simulink model "Leg_Sim_VariableDamping"  (R2020b)
settings: Solver=ode23s  StartTime=0.0  StopTime=1  RelTol=1e-3
values from neighbouring files (symbols this model uses):
  body = Leg_Pars_Body    [Leg_Script_Powered.m]    (also in Leg_Script_Socket_VariableDamping.m; Leg_Script_VariableDamping.m)
  ctrl = Leg_Pars_Ctrl_Powered    [Leg_Script_Powered.m]    (also in Leg_Script_Socket_VariableDamping.m = Leg_Pars_Ctrl_VariableDamping; Leg_Script_VariableDamping.m = Leg_Pars_Ctrl_VariableDamping)
  device = Leg_Pars_Device_Powered    [Leg_Script_Powered.m]    (also in Leg_Script_Socket_VariableDamping.m = Leg_Pars_Device_VariableDamping; Leg_Script_VariableDamping.m = Leg_Pars_Device_VariableDamping)
  FD = [1;1;0;1;1;0;0;1]    [Leg_Script_Powered.m]    (also in Leg_Script_Socket_VariableDamping.m = [1;1;0;1;1;1;1;0;0;1]; Leg_Script_VariableDamping.m)
  human = Leg_Pars_Human(body)    [Leg_Script_Powered.m]    (also in Leg_Script_Socket_VariableDamping.m; Leg_Script_VariableDamping.m)
  intent = [0;1;0]    [Leg_Script_Powered.m]    (also in Leg_Script_Socket_VariableDamping.m; Leg_Script_VariableDamping.m)
  intentv = [1.1;1.1;0.8]    [Leg_Script_Powered.m]    (also in Leg_Script_Socket_VariableDamping.m = [1.1; 1.1; 1.4; 1.4; 1.1; 1.1; 1.4;0.8]; Leg_Script_VariableDamping.m = [1.1; 1.1; 1.4; 1.4; 1.1; 1.1; 1.4;0.8])
  q0 = [0;1;ref.pt_walk ... (first row only)    [Leg_Script_Powered.m]    (also in Leg_Script_Socket_VariableDamping.m; Leg_Script_VariableDamping.m)
  qd0 = [intentv(1)*1.2*intent(1);0;0;0;0;0;0;0]    [Leg_Script_Powered.m]    (also in Leg_Script_Socket_VariableDamping.m = [intentv(1)*1.25*intent(1);0;0;0;0;0;0;0;0;0]; Leg_Script_VariableDamping.m)
  robsim = robotcell2mat(robot)    [Leg_Script_Powered.m]    (also in Leg_Script_Socket_VariableDamping.m; Leg_Script_VariableDamping.m)
  t_intent = [0;1;15]    [Leg_Script_Powered.m]    (also in Leg_Script_Socket_VariableDamping.m = [0;1;35]; Leg_Script_VariableDamping.m = [0;1;35])
  t_intentv = [0;10;15]    [Leg_Script_Powered.m]    (also in Leg_Script_Socket_VariableDamping.m = [0; 9.99; 10; 14.99; 15; 20; 25;35]; Leg_Script_VariableDamping.m = [0; 9.99; 10; 14.99; 15; 20; 25;35])
  u0 = zeros(1,length(robot.gc.body))    [Leg_Script_Powered.m]    (also in Leg_Script_Socket_VariableDamping.m; Leg_Script_VariableDamping.m)
undefined symbols (not defined in the file or in its folder): syst
libraries: simulink x4
(part 1 of 2)
settings Model: Creator=JDriessen  LastModifiedBy=jdriessen
settings SolverCC: ZeroCrossAlgorithm=Adaptive
settings DebuggingCC: MaskedZcDiagnostic=none  IgnoredZcDiagnostic=none

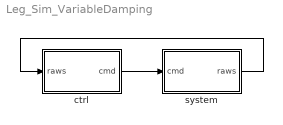
== system Leg_Sim_VariableDamping ==
  ctrl : Subsystem
  system : Subsystem
  wires:
  system/1(raws) -> ctrl/1(raws)
  ctrl/1(cmd) -> system/1(cmd)

== system Leg_Sim_VariableDamping/ctrl ==
  raws : Inport
  Clock : Clock
      settings: Decimation=3
  High-level ctrl : Subsystem  mask{fsm=ctrl.fsm}
      mask prompts: fsm "FSM Parameters"
      mask help: High-level control: Finite State Machine (FSM)
  Mid-level ctrl : Subsystem  mask{mid=ctrl.mid}
      mask prompts: mid "Mid-level controller parameters"
      mask help: Mid-level control
      mask DialogControl Container2 Prompt: Parameters
  Signal processing : Subsystem  mask{pre=ctrl.pre}
      mask prompts: pre "Signal processing parameters"
      mask help: Signal processing
  clock : ToWorkspace  VariableName=t_ctrl  SampleTime=ctrl.t_step
      settings: Save2DSignal=2-D array (concatenate along first dimension)
  cmd : Outport
  wires:
  raws/1 -> Signal processing/1(raws)
  Mid-level ctrl/1(cmd) -> cmd/1
  High-level ctrl/1(state) -> Mid-level ctrl/2(state)
  Clock/1 -> clock/1
  Signal processing/2(tube) -> High-level ctrl/2(tube)
  Signal processing/1(knee) -> High-level ctrl/1(knee), Mid-level ctrl/1(knee)

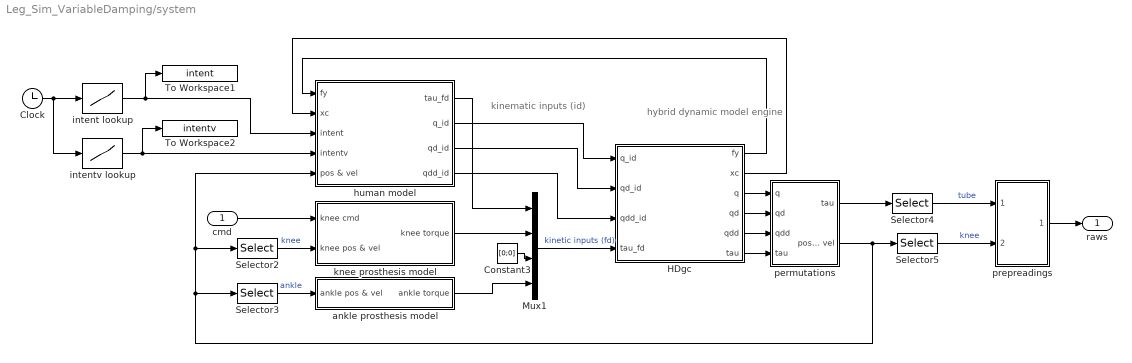
== system Leg_Sim_VariableDamping/system ==
  note: kinematic inputs (id)
  note: hybrid dynamic
      | model engine
  cmd : Inport
  Clock : Clock
  Constant3 : Constant  Value=[0;0]
  HDgc : Subsystem  mask{model=robsim, fd=FD, q0=q0, qd0=qd0, u0=u0}
      mask prompts: model "robot structure"; fd "joint dynamics type logic (1=forward, 0=inverse)"; q0 "initial joint position (forward dynamics)"; qd0 "initial joint velocities (forward dynamics)"; u0 "initial ground contact deformations"
      mask help: Hybrid dynamics engine with ground contact model.
      mask init:
      | fdd = fd~=0; % convert to logical (if not already)
      | i_fd = find(fd); % indices fd joints
      | model.fd_i = cumsum(fd); % joint index assign array fd joints
      | model.NB_fd = sum(fd); % number of fd joints
      | i_id = find(~fd); % indices id joints
      | model.id_i = cumsum(~fd); % joint index assign array id joints
      | model.NB_id = sum(~fd); % number of id joints
      | model.ND = size(model.Xtree(:,:,1),1); % 3 = planar, 6 = spatial
      | model.S = zeros(model.ND,model.NB); % pre-allocate motion subspace matrix
      | for i = 1:model.NB % fill motion subspace matrix
      |     switch model.jtype(i,:)
      |     case 'Rx' % revolute X axis
      |         model.S = [1;0;0;0;0;0];
      |     case 'Ry' % revolute Y axis
      |         model.S = [0;1;0;0;0;0];
      |     case 'Rz' % revolute Z axis
      |         model.S = [0;0;1;0;0;0];
      |     case 'Px' % prismatic X axis
      |         model.S = [0;0;0;1;0;0];
      |     case 'Py' % prismatic Y axis
      |         model.S = [0;0;0;0;1;0];
      |     case 'Pz' % prismatic Z axis
      |         model.S = [0;0;0;0;0;1];
      |     case 'Hz' % helical (Z axis)
      |         model.S = [0;0;1;0;0;jtyp.pars.pitch];
      |     case 'rz' % planar revolute
      |         model.S(:,i) = [1;0;0];
      |     case 'px'% planar prismatic X axis
      |         model.S(:,i) = [0;1;0];
      |     case 'py'% planar prismatic Y axis
      |         model.S(:,i) = [0;0;1];
      |     otherwise
      |         error( 'unrecognised joint code ''%s''', code );
      |     end
      | end
      | % gravity
      | g = model.gravity;
      | if model.ND == 3		% is model planar?
      |     model.a_grav = [0;g(1);g(2)];
      | else
      |     model.a_grav = [0;0;0;g(1);g(2);g(3)];
      | end
  Mux1 : Mux
  Selector2 : Selector  InputPortWidth=robsim.NB*2  IndexOptions=Index vector (dialog)  Indices=5+[0;robsim.NB]  OutputSizes=1
  Selector3 : Selector  InputPortWidth=robsim.NB*2  IndexOptions=Index vector (dialog)  Indices=8+[0;robsim.NB]  OutputSizes=1
  Selector4 : Selector  InputPortWidth=robsim.NB  IndexOptions=Index vector (dialog)  Indices=[7;6]  OutputSizes=1
  Selector5 : Selector  InputPortWidth=robsim.NB*2  IndexOptions=Index vector (dialog)  Indices=5  OutputSizes=1
  To Workspace1 : ToWorkspace  VariableName=intent  SampleTime=-1
      settings: Save2DSignal=2-D array (concatenate along first dimension)
  To Workspace2 : ToWorkspace  VariableName=intentv  SampleTime=-1
      settings: Save2DSignal=2-D array (concatenate along first dimension)
  ankle prosthesis model : Subsystem  mask{ank=device.ankle}
      mask prompts: ank "ankle parameters"
      mask help: Ankle Prosthesis Model
  human model : Subsystem  mask{ref=human.ref, imp=human.imp, SLIP=human.SLIP, x_step_0=human.x_step_0, Kthrust_0=human.Kthrust_0, bdy=body, rob=robsim}
      mask prompts: ref "human reference trajectories and parameters"; imp "human impedance parameters"; SLIP "human SLIP parameters"; x_step_0 "initial estimate step length"; Kthrust_0 "initial estimate thrust gain"; bdy "body parameters"; rob "robot structure"
      mask help: Human model
  intent lookup : Lookup_n-D  NumberOfTableDimensions=1  BreakpointsForDimension1=t_intent  IndexSearchMethod=Linear search  Table=intent  InterpMethod=Flat  InternalRulePriority=Speed  RndMeth=Simplest  InputSameDT=on
  intentv lookup : Lookup_n-D  NumberOfTableDimensions=1  BreakpointsForDimension1=t_intentv  IndexSearchMethod=Linear search  Table=intentv  ExtrapMethod=Clip  InternalRulePriority=Speed  RndMeth=Simplest  InputSameDT=on
  knee prosthesis model : Subsystem  mask{dmp=device.knee.damper, ese=device.knee.ext_endstop, esf=device.knee.flx_endstop}
      mask prompts: dmp "knee damper parameters"; ese "knee extension endstop parameters"; esf "knee flexion endstop parameters"
      mask help: Knee Prosthesis Model
  permutations : Subsystem
  prepreadings : Subsystem
  raws : Outport
  wires:
  Mux1/1 -> HDgc/4(tau_fd)  "kinetic inputs (fd)"
  Selector5/1 -> prepreadings/2(knee pos)  "knee"
  Selector4/1 -> prepreadings/1(tube)  "tube"
  Constant3/1 -> Mux1/3
  cmd/1 -> knee prosthesis model/1(knee cmd)
  Selector2/1 -> knee prosthesis model/2(knee pos & vel)  "knee"
  knee prosthesis model/1(knee torque) -> Mux1/2
  Selector3/1 -> ankle prosthesis model/1(ankle pos & vel)  "ankle"
  ankle prosthesis model/1(ankle torque) -> Mux1/4
  HDgc/3(q) -> permutations/1(q)
  HDgc/6(tau) -> permutations/4("tau ")
  permutations/1(tau) -> Selector4/1
  prepreadings/1(raws) -> raws/1
  intent lookup/1 -> human model/3(intent), To Workspace1/1
  permutations/2(pos & vel) -> human model/5(pos & vel), Selector2/1, Selector3/1, Selector5/1
  Clock/1 -> intentv lookup/1, intent lookup/1
  intentv lookup/1 -> human model/4(intentv), To Workspace2/1
  human model/4(qdd_id) -> HDgc/3(qdd_id)
  human model/3(qd_id) -> HDgc/2(qd_id)
  human model/2(q_id) -> HDgc/1(q_id)
  human model/1(tau_fd) -> Mux1/1
  HDgc/1(fy) -> human model/1(fy)
  HDgc/2(xc) -> human model/2(xc)
  HDgc/4(qd) -> permutations/2(qd)
  HDgc/5(qdd) -> permutations/3(qdd)

== system Leg_Sim_VariableDamping/ctrl/High-level ctrl ==
  knee : Inport
  tube : Inport  Port=2
  Chart : Stateflow chart  TreatAsAtomicUnit=on
  Demux : Demux  Outputs=2
  Demux1 : Demux  Outputs=2
  To Workspace : ToWorkspace  VariableName=state  SampleTime=ctrl.t_step
      settings: Save2DSignal=2-D array (concatenate along first dimension)
  To Workspace1 : ToWorkspace  VariableName=tSt  SampleTime=-1
      settings: Save2DSignal=2-D array (concatenate along first dimension)
  To Workspace2 : ToWorkspace  VariableName=tSw  SampleTime=-1
      settings: Save2DSignal=2-D array (concatenate along first dimension)
  state : Outport
  wires:
  Chart/1(state) -> To Workspace/1, state/1
  Demux/2 -> Chart/2(wk)  "pkd"
  Demux/1 -> Chart/1(pk)  "pk"
  knee/1 -> Demux/1
  tube/1 -> Demux1/1
  Demux1/1 -> Chart/3(M)
  Chart/2(tSw) -> To Workspace2/1
  Chart/3(tSt) -> To Workspace1/1
  Demux1/2 -> Chart/4(F)  "F"

== system Leg_Sim_VariableDamping/ctrl/Mid-level ctrl ==
  knee : Inport
  state : Inport  Port=2
  Demux1 : Demux  Outputs=2
  Mid Ctrl : MATLAB Function  Description=Mid-level control  TreatAsAtomicUnit=on  SystemSampleTime=ctrl.t_step
  Terminator2 : Terminator
  To Workspace2 : ToWorkspace  VariableName=cmd_m  SampleTime=-1
      settings: Save2DSignal=2-D array (concatenate along first dimension)
  cmd : Outport
  wires:
  Mid Ctrl/1(cmd_m) -> To Workspace2/1, cmd/1
  state/1 -> Mid Ctrl/2(state)
  knee/1 -> Demux1/1
  Demux1/1 -> Mid Ctrl/1(pk)  "pk"
  Demux1/2 -> Terminator2/1  "pkd"

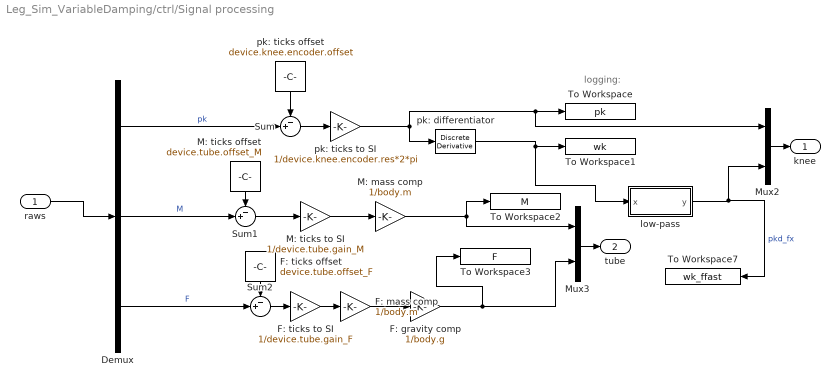
== system Leg_Sim_VariableDamping/ctrl/Signal processing ==
  note: logging:
  raws : Inport
  Demux : Demux  Outputs=3
  F: gravity comp : Gain  Gain=1/body.g
  F: mass comp : Gain  Gain=1/body.m
  F: ticks offset : Constant  Value=device.tube.offset_F
  F: ticks to SI : Gain  Gain=1/device.tube.gain_F
  M: mass comp : Gain  Gain=1/body.m
  M: ticks offset : Constant  Value=device.tube.offset_M
  M: ticks to SI : Gain  Gain=1/device.tube.gain_M
  Mux2 : Mux  Inputs=2
  Mux3 : Mux  Inputs=2
  Sum : Sum  Inputs=-+|
  Sum1 : Sum  Inputs=-+|
  Sum2 : Sum  Inputs=-+|
  To Workspace : ToWorkspace  VariableName=pk  SampleTime=-1
      settings: Save2DSignal=2-D array (concatenate along first dimension)
  To Workspace1 : ToWorkspace  VariableName=wk  SampleTime=-1
      settings: Save2DSignal=2-D array (concatenate along first dimension)
  To Workspace2 : ToWorkspace  VariableName=M  SampleTime=-1
      settings: Save2DSignal=2-D array (concatenate along first dimension)
  To Workspace3 : ToWorkspace  VariableName=F  SampleTime=-1
      settings: Save2DSignal=2-D array (concatenate along first dimension)
  To Workspace7 : ToWorkspace  VariableName=wk_ffast  SampleTime=-1
      settings: Save2DSignal=2-D array (concatenate along first dimension)
  low-pass : Subsystem  mask(1st order Butterworth filter){Wn=pre.freq_fast*ctrl.t_step*2, x0=0, y0=0}
      mask prompts: Wn "cut-off frequency"; x0 "initial condition for previous input"; y0 "initial condition for previous output"
      mask help: The cut-off frequency Wn must be 0.0 < Wn < 1.0, with 1.0 corresponding to half the sample rate.
  pk: differentiator : simulink/Discrete/Discrete Derivative  gainval=1  ICPrevScaledInput=0  OutMin=[]  OutMax=[]  OutDataType=fixdt(1, 16)  OutScaling=2^-10  DoSatur=off
  pk: ticks offset : Constant  Value=device.knee.encoder.offset
  pk: ticks to SI : Gain  Gain=1/device.knee.encoder.res*2*pi
  knee : Outport
  tube : Outport  Port=2
  wires:
  F: gravity comp/1 -> To Workspace3/1, Mux3/2
  F: ticks to SI/1 -> F: mass comp/1
  low-pass/1(y) -> Mux2/2, To Workspace7/1  "pkd_fx"
  Mux3/1 -> tube/1
  pk: ticks to SI/1 -> Mux2/1, To Workspace/1, pk: differentiator/1
  F: mass comp/1 -> F: gravity comp/1
  pk: differentiator/1 -> low-pass/1(x), To Workspace1/1
  M: mass comp/1 -> To Workspace2/1, Mux3/1
  Mux2/1 -> knee/1
  Sum2/1 -> F: ticks to SI/1
  raws/1 -> Demux/1
  F: ticks offset/1 -> Sum2/1
  M: ticks to SI/1 -> M: mass comp/1
  M: ticks offset/1 -> Sum1/1
  Sum/1 -> pk: ticks to SI/1
  Sum1/1 -> M: ticks to SI/1
  pk: ticks offset/1 -> Sum/1
  Demux/1 -> Sum/2  "pk"
  Demux/2 -> Sum1/2  "M"
  Demux/3 -> Sum2/2  "F"

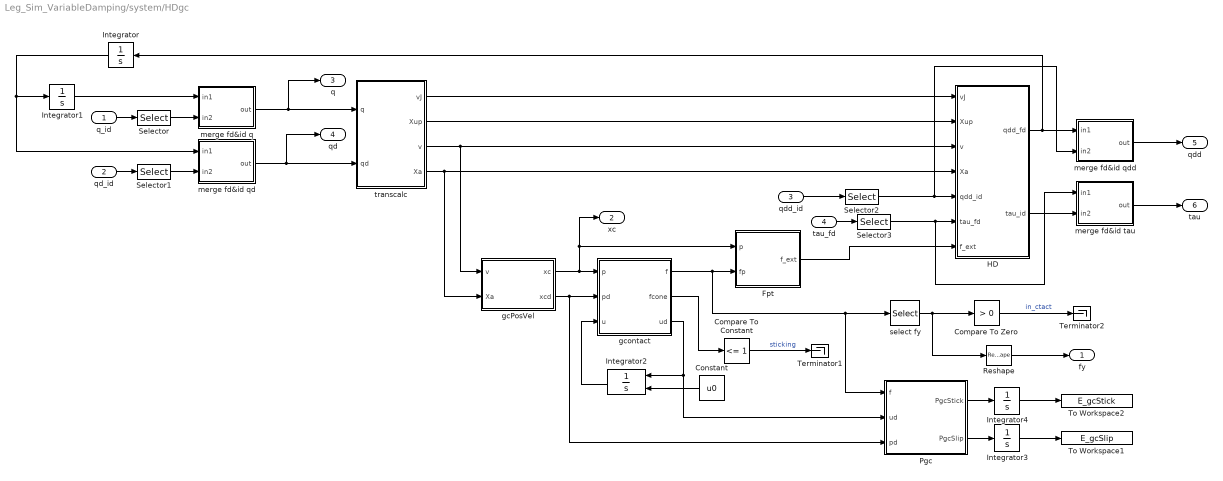
== system Leg_Sim_VariableDamping/system/HDgc ==
  q_id : Inport
  qd_id : Inport  Port=2
  qdd_id : Inport  Port=3
  tau_fd : Inport  Port=4
  Compare To Constant : simulink/Logic and Bit Operations/Compare To Constant  relop=<=  const=1  OutDataTypeStr=boolean
  Compare To Zero : simulink/Logic and Bit Operations/Compare To Zero  relop=>  OutDataTypeStr=boolean
  Constant : Constant  Value=u0  VectorParams1D=off
  Fpt : MATLAB Function  TreatAsAtomicUnit=on
  HD : MATLAB Function  TreatAsAtomicUnit=on
  Integrator : Integrator  InitialCondition=qd0(i_fd)
  Integrator1 : Integrator  InitialCondition=q0(i_fd)
  Integrator2 : Integrator  InitialConditionSource=external  InitialCondition=syst.u0
  Integrator3 : Integrator
  Integrator4 : Integrator
  Pgc : MATLAB Function  TreatAsAtomicUnit=on
  Reshape : Reshape
  Selector : Selector  InputPortWidth=model.NB  IndexOptions=Index vector (dialog)  Indices=i_id  OutputSizes=1
  Selector1 : Selector  InputPortWidth=model.NB  IndexOptions=Index vector (dialog)  Indices=i_id  OutputSizes=1
  Selector2 : Selector  InputPortWidth=model.NB  IndexOptions=Index vector (dialog)  Indices=i_id  OutputSizes=1
  Selector3 : Selector  InputPortWidth=model.NB  IndexOptions=Index vector (dialog)  Indices=i_fd  OutputSizes=1
  Terminator1 : Terminator
  Terminator2 : Terminator
  To Workspace1 : ToWorkspace  VariableName=E_gcSlip  SampleTime=-1
      settings: Save2DSignal=2-D array (concatenate along first dimension)
  To Workspace2 : ToWorkspace  VariableName=E_gcStick  SampleTime=-1
      settings: Save2DSignal=2-D array (concatenate along first dimension)
  gcPosVel : MATLAB Function  TreatAsAtomicUnit=on
  gcontact : MATLAB Function  TreatAsAtomicUnit=on
  merge fd&id q : Subsystem  mask(Merge Assignment){}
      mask help: Merges two input arrays IN1 and IN2 into a single output array OUT according to assignment array FD, where elements of IN1 and IN2 are assigned to elements of OUT sequentially for which elements of FD are true and false respectively. FD must be defined to that length(FD) = length(OUT) = length(IN1) + length(IN2), sum(FD) = length(IN1), and sum(~FD)=length(IN2).
  merge fd&id qd : Subsystem  mask(Merge Assignment){}
      mask help: Merges two input arrays IN1 and IN2 into a single output array OUT according to assignment array FD, where elements of IN1 and IN2 are assigned to elements of OUT sequentially for which elements of FD are true and false respectively. FD must be defined to that length(FD) = length(OUT) = length(IN1) + length(IN2), sum(FD) = length(IN1), and sum(~FD)=length(IN2).
  merge fd&id qdd : Subsystem  mask(Merge Assignment){}
      mask help: Merges two input arrays IN1 and IN2 into a single output array OUT according to assignment array FD, where elements of IN1 and IN2 are assigned to elements of OUT sequentially for which elements of FD are true and false respectively. FD must be defined to that length(FD) = length(OUT) = length(IN1) + length(IN2), sum(FD) = length(IN1), and sum(~FD)=length(IN2).
  merge fd&id tau : Subsystem  mask(Merge Assignment){}
      mask help: Merges two input arrays IN1 and IN2 into a single output array OUT according to assignment array FD, where elements of IN1 and IN2 are assigned to elements of OUT sequentially for which elements of FD are true and false respectively. FD must be defined to that length(FD) = length(OUT) = length(IN1) + length(IN2), sum(FD) = length(IN1), and sum(~FD)=length(IN2).
  select fy : Selector  NumberOfDimensions=2  InputPortWidth=3  IndexOptions=Index vector (dialog),Select all  Indices=[2],1  OutputSizes=1,1
  transcalc : MATLAB Function  TreatAsAtomicUnit=on
  fy : Outport
  xc : Outport  Port=2
  q : Outport  Port=3
  qd : Outport  Port=4
  qdd : Outport  Port=5
  tau : Outport  Port=6
  wires:
  Integrator/1 -> merge fd&id qd/1(in1), Integrator1/1
  qd_id/1 -> Selector1/1
  transcalc/3(v) -> gcPosVel/1(v), HD/3(v)
  transcalc/4(Xa) -> gcPosVel/2(Xa), HD/4(Xa)
  gcPosVel/1(xc) -> xc/1, Fpt/1(p), gcontact/1(p)
  gcPosVel/2(xcd) -> gcontact/2(pd), Pgc/3(pd)
  gcontact/3(ud) -> Pgc/2(ud), Integrator2/1
  Integrator2/1 -> gcontact/3(u)
  Constant/1 -> Integrator2/2
  select fy/1 -> Reshape/1, Compare To Zero/1
  gcontact/2(fcone) -> Compare To Constant/1
  Compare To Zero/1 -> Terminator2/1  "in_ctact"
  gcontact/1(f) -> Pgc/1(f), select fy/1, Fpt/2(fp)
  Integrator3/1 -> To Workspace1/1
  Pgc/2(PgcSlip) -> Integrator3/1
  Integrator4/1 -> To Workspace2/1
  Pgc/1(PgcStick) -> Integrator4/1
  Compare To Constant/1 -> Terminator1/1  "sticking"
  transcalc/1(vJ) -> HD/1(vJ)
  Fpt/1(f_ext) -> HD/7(f_ext)
  tau_fd/1 -> Selector3/1
  qdd_id/1 -> Selector2/1
  transcalc/2(Xup) -> HD/2(Xup)
  Selector/1 -> merge fd&id q/2(in2)
  q_id/1 -> Selector/1
  Selector1/1 -> merge fd&id qd/2(in2)
  merge fd&id q/1(out) -> q/1, transcalc/1(q)
  merge fd&id qd/1(out) -> qd/1, transcalc/2(qd)
  merge fd&id tau/1(out) -> tau/1
  Selector2/1 -> merge fd&id qdd/2(in2), HD/5(qdd_id)
  Selector3/1 -> merge fd&id tau/1(in1), HD/6(tau_fd)
  HD/1(qdd_fd) -> Integrator/1, merge fd&id qdd/1(in1)
  Integrator1/1 -> merge fd&id q/1(in1)
  HD/2(tau_id) -> merge fd&id tau/2(in2)
  merge fd&id qdd/1(out) -> qdd/1
  Reshape/1 -> fy/1

== system Leg_Sim_VariableDamping/system/ankle prosthesis model ==
  ankle pos & vel : Inport
  Demux3 : Demux  Outputs=2
  To Workspace12 : ToWorkspace  VariableName=E_ankle  SampleTime=-1
      settings: Save2DSignal=2-D array (concatenate along first dimension)
  spring damper : Subsystem
  ankle torque : Outport
  wires:
  Demux3/1 -> spring damper/1(x)  "q8"
  spring damper/1(F) -> ankle torque/1
  spring damper/2(E) -> To Workspace12/1
  Demux3/2 -> spring damper/2(xd)  "q8d"
  ankle pos & vel/1 -> Demux3/1

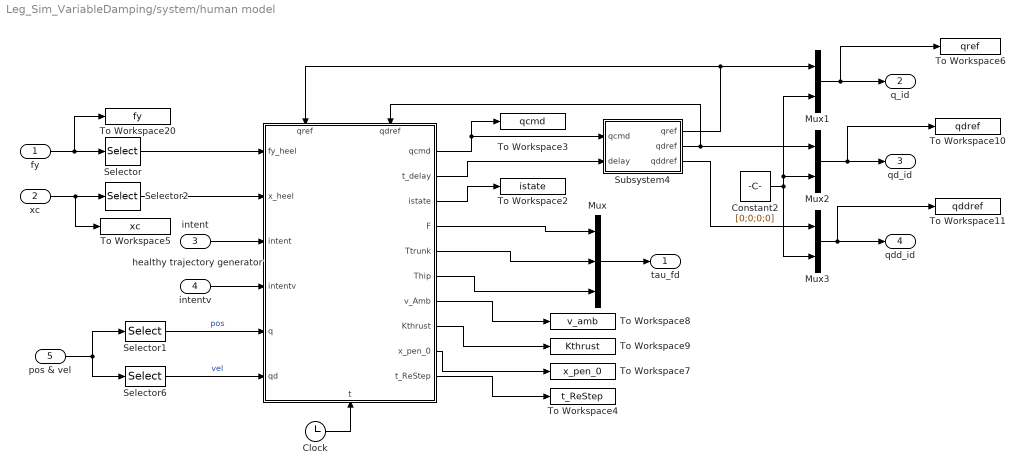
== system Leg_Sim_VariableDamping/system/human model ==
  fy : Inport
  xc : Inport  Port=2
  intent : Inport  Port=3
  intentv : Inport  Port=4
  pos & vel : Inport  Port=5
  Clock : Clock
  Constant2 : Constant  Value=[0;0;0;0]
  Mux : Mux  Inputs=3
  Mux1 : Mux  Inputs=2
  Mux2 : Mux  Inputs=2
  Mux3 : Mux  Inputs=2
  Selector : Selector  InputPortWidth=length(rob.gc.body)  IndexOptions=Index vector (dialog)  Indices=5  OutputSizes=1
  Selector1 : Selector  InputPortWidth=rob.NB*2  IndexOptions=Index vector (dialog)  Indices=[1:rob.NB]  OutputSizes=1
  Selector2 : Selector  NumberOfDimensions=2  InputPortWidth=6  IndexOptions=Index vector (dialog),Index vector (dialog)  Indices=1,5  OutputSizes=1,1
  Selector6 : Selector  InputPortWidth=rob.NB*2  IndexOptions=Index vector (dialog)  Indices=[rob.NB+1:rob.NB*2]  OutputSizes=1
  Subsystem4 : Subsystem
  To Workspace10 : ToWorkspace  VariableName=qdref  SampleTime=-1
      settings: Save2DSignal=2-D array (concatenate along first dimension)
  To Workspace11 : ToWorkspace  VariableName=qddref  SampleTime=-1
      settings: Save2DSignal=2-D array (concatenate along first dimension)
  To Workspace2 : ToWorkspace  VariableName=istate  SampleTime=-1
      settings: Save2DSignal=2-D array (concatenate along first dimension)
  To Workspace20 : ToWorkspace  VariableName=fy  SampleTime=-1
      settings: Save2DSignal=2-D array (concatenate along first dimension)
  To Workspace3 : ToWorkspace  VariableName=qcmd  SampleTime=-1
      settings: Save2DSignal=2-D array (concatenate along first dimension)
  To Workspace4 : ToWorkspace  VariableName=t_ReStep  SampleTime=-1
      settings: Save2DSignal=2-D array (concatenate along first dimension)
  To Workspace5 : ToWorkspace  VariableName=xc  SampleTime=-1
  To Workspace6 : ToWorkspace  VariableName=qref  SampleTime=-1
      settings: Save2DSignal=2-D array (concatenate along first dimension)
  To Workspace7 : ToWorkspace  VariableName=x_pen_0  SampleTime=-1
      settings: Save2DSignal=2-D array (concatenate along first dimension)
  To Workspace8 : ToWorkspace  VariableName=v_amb  SampleTime=-1
      settings: Save2DSignal=2-D array (concatenate along first dimension)
  To Workspace9 : ToWorkspace  VariableName=Kthrust  SampleTime=-1
      settings: Save2DSignal=2-D array (concatenate along first dimension)
  healthy trajectory generator : Stateflow chart  TreatAsAtomicUnit=on
      settings: PortSchema="{\"entries\":[{\"content\":{\"sides\":[{\"content\":{\"connectorIds\":[\"In1\",\"In2\",\"In3\",\"In4\",\"In5\",\"In6\"]},\"type\":\"ConnectorPlacement.EquallySpacedRectSide\",\"uuid\":\"f082dfa6-a80b-4b96-9ecb-6cbc0012c766\"},{\"content\":{\"connectorIds\":[\"Out1\",\"Out2\",\"Out3\",\"Out4\",\"Out5\",\"Out6\",\"Out7\",\"Out8\",\"Out9\",\"Out10\"],\"side\":\"RIGHT\"},\"type\":\"ConnectorPlacement.EquallySpacedRectSide\",\"uuid\":\"95252e94-213a-4b45-aa38-ebc7e45d4671\"},{\"content\":{\"connectorIds\":[\"In7\",\"In8\"],\"side\":\"TOP\"},\"type\":\"ConnectorPlacement.EquallySpacedRectSide\",\"uuid\":\"2e5ad652-03a7-4ead-9149-801c25da5955\"},{\"content\":{\"connectorIds\":[\"In9\"],\"side\":\"BOTTOM\"},\"type\":\"ConnectorPlacement.EquallySpacedRectSide\",\"uuid\":\"8173bb4b-d730-47f7-871f-e7c876bfac20\"},{\"content\":{\"connectorIds\":[],\"side\":\"HIDDEN\"},\"type\":\"ConnectorPlacement.EquallySpacedRectSide\",\"uuid\":\"61de4bae-a869-42e5-a778-93a8d5d6640c\"}]},\"type\":\"ConnectorPlacement.EquallySpacedConnector\",\"uuid\":\"f5308c7a-89dd-4e9c-9b64-0a9b2194fc69\"}],\"packageUris\":[\"http://schema.mathworks.com/mf0/Connector/R2020b\"],\"version\":\"1.0\"}"
  tau_fd : Outport
  q_id : Outport  Port=2  PortDimensions=rob.NB
  qd_id : Outport  Port=3  PortDimensions=rob.NB
  qdd_id : Outport  Port=4  PortDimensions=rob.NB
  wires:
  Mux/1 -> tau_fd/1
  fy/1 -> Selector/1, To Workspace20/1
  intent/1 -> healthy trajectory generator/3(intent)
  Selector6/1 -> healthy trajectory generator/6(qd)  "vel"
  Selector1/1 -> healthy trajectory generator/5(q)  "pos"
  pos & vel/1 -> Selector6/1, Selector1/1
  healthy trajectory generator/3(istate) -> To Workspace2/1
  xc/1 -> To Workspace5/1, Selector2/1
  Selector2/1 -> healthy trajectory generator/2(x_heel)
  intentv/1 -> healthy trajectory generator/4(intentv)
  healthy trajectory generator/4(F) -> Mux/1
  healthy trajectory generator/6(Thip) -> Mux/3
  healthy trajectory generator/5(Ttrunk) -> Mux/2
  healthy trajectory generator/9(x_pen_0) -> To Workspace7/1
  healthy trajectory generator/7(v_Amb) -> To Workspace8/1
  healthy trajectory generator/8(Kthrust) -> To Workspace9/1
  healthy trajectory generator/1(qcmd) -> Subsystem4/1(qcmd), To Workspace3/1
  healthy trajectory generator/2(t_delay) -> Subsystem4/2(delay)
  Subsystem4/1(qref) -> Mux1/1, healthy trajectory generator/7(qref)
  Subsystem4/2(qdref) -> Mux2/1, healthy trajectory generator/8(qdref)
  Subsystem4/3(qddref) -> Mux3/1
  Constant2/1 -> Mux1/2, Mux2/2, Mux3/2
  Mux1/1 -> To Workspace6/1, q_id/1
  Mux2/1 -> To Workspace10/1, qd_id/1
  Mux3/1 -> To Workspace11/1, qdd_id/1
  healthy trajectory generator/10(t_ReStep) -> To Workspace4/1
  Selector/1 -> healthy trajectory generator/1(fy_heel)
  Clock/1 -> healthy trajectory generator/9(t)

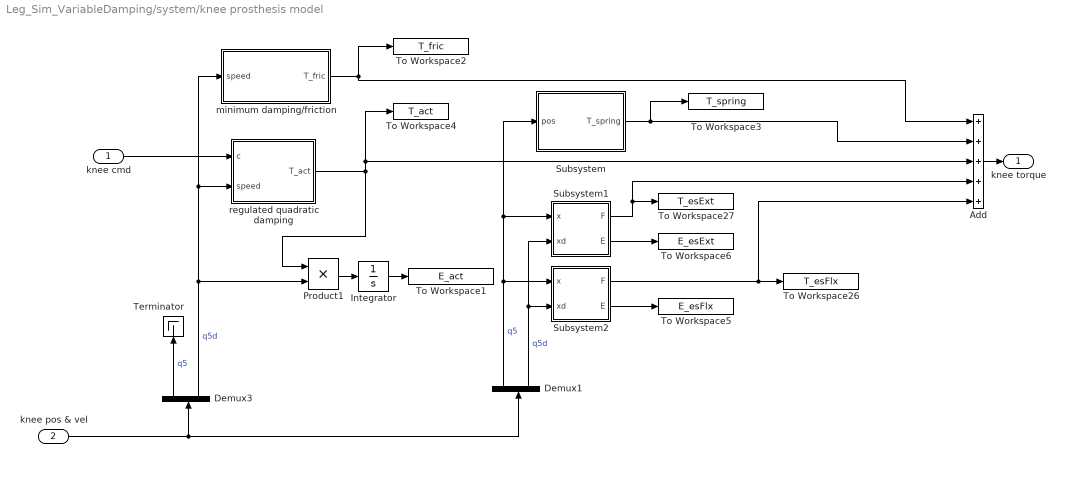
== system Leg_Sim_VariableDamping/system/knee prosthesis model ==
  knee cmd : Inport
  knee pos & vel : Inport  Port=2
  Add : Sum  Inputs=+++++
  Demux1 : Demux  Outputs=2
  Demux3 : Demux  Outputs=2
  Integrator : Integrator
  Product1 : Product
  Subsystem : Subsystem
  Subsystem1 : Subsystem  mask(Compliant End Stop){dir=upper limit, pos=-ese.p_0, F=ese.T_half, d=ese.p_tot, tc=ese.t_c}
      mask prompts: dir "Type of End Stop"; pos "Position of End Stop (place at which it begins to operate)"; F "Force or Torque at a compression of half the thickness [N or Nm]"; d "Thickness [m or rad]"; tc "Recovery Time Constant [s]"
      mask help: Compliant end stop with nonlinear stiffness and damping. INPUTS: position and velocity variables affected by the end stop (x and xd). OUTPUTS: force produced by the end stop (F), measured in the same sense as x (so F>0 for a lower-limit end stop) and bus (E) containing the power and energy signals for an energy audit. As the stiffness and damping are nonlinear, you specify a desired static force at a compression of half the endstop thickness and a desired recovery time constant. The bigger the time constant, the less bouncy the end stop. Formula: F=2/7*(K*(x/d-(d/x)^2)+D*(xd/d)*(1+2*(d/x)^3)))
      mask TypeOptions dir: lower limit | upper limit
      mask Display: disp('Finite\nEnd\nStop')
  Subsystem2 : Subsystem  mask(Compliant End Stop){dir=lower limit, pos=-esf.p_0, F=ese.T_half, d=esf.p_tot, tc=esf.t_c}
      mask prompts: dir "Type of End Stop"; pos "Position of End Stop (place at which it begins to operate)"; F "Force or Torque at a compression of half the thickness [N or Nm]"; d "Thickness [m or rad]"; tc "Recovery Time Constant [s]"
      mask help: Compliant end stop with nonlinear stiffness and damping. INPUTS: position and velocity variables affected by the end stop (x and xd). OUTPUTS: force produced by the end stop (F), measured in the same sense as x (so F>0 for a lower-limit end stop) and bus (E) containing the power and energy signals for an energy audit. As the stiffness and damping are nonlinear, you specify a desired static force at a compression of half the endstop thickness and a desired recovery time constant. The bigger the time constant, the less bouncy the end stop. Formula: F=2/7*(K*(x/d-(d/x)^2)+D*(xd/d)*(1+2*(d/x)^3)))
      mask TypeOptions dir: lower limit | upper limit
      mask Display: disp('Finite\nEnd\nStop')
  Terminator : Terminator
  To Workspace1 : ToWorkspace  VariableName=E_act  SampleTime=-1
      settings: Save2DSignal=2-D array (concatenate along first dimension)
  To Workspace2 : ToWorkspace  VariableName=T_fric  SampleTime=-1
      settings: Save2DSignal=2-D array (concatenate along first dimension)
  To Workspace26 : ToWorkspace  VariableName=T_esFlx  SampleTime=-1
      settings: Save2DSignal=2-D array (concatenate along first dimension)
  To Workspace27 : ToWorkspace  VariableName=T_esExt  SampleTime=-1
      settings: Save2DSignal=2-D array (concatenate along first dimension)
  To Workspace3 : ToWorkspace  VariableName=T_spring  SampleTime=-1
      settings: Save2DSignal=2-D array (concatenate along first dimension)
  To Workspace4 : ToWorkspace  VariableName=T_act  SampleTime=-1
      settings: Save2DSignal=2-D array (concatenate along first dimension)
  To Workspace5 : ToWorkspace  VariableName=E_esFlx  SampleTime=-1
      settings: Save2DSignal=2-D array (concatenate along first dimension)
  To Workspace6 : ToWorkspace  VariableName=E_esExt  SampleTime=-1
      settings: Save2DSignal=2-D array (concatenate along first dimension)
  minimum damping/friction : Subsystem
  regulated quadratic damping : Subsystem
  knee torque : Outport
  wires:
  Demux1/2 -> Subsystem1/2(xd), Subsystem2/2(xd)  "q5d"
  Subsystem1/2(E) -> To Workspace6/1
  Demux1/1 -> Subsystem2/1(x), Subsystem/1(pos), Subsystem1/1(x)  "q5"
  Add/1 -> knee torque/1
  Subsystem1/1(F) -> Add/4, To Workspace27/1
  Subsystem2/2(E) -> To Workspace5/1
  Subsystem2/1(F) -> Add/5, To Workspace26/1
  Product1/1 -> Integrator/1
  Integrator/1 -> To Workspace1/1
  Demux3/2 -> minimum damping/friction/1(speed), regulated quadratic damping/2(speed), Product1/2  "q5d"
  regulated quadratic damping/1(T_act) -> Add/3, To Workspace4/1, Product1/1
  Demux3/1 -> Terminator/1  "q5"
  knee cmd/1 -> regulated quadratic damping/1(c)
  minimum damping/friction/1(T_fric) -> To Workspace2/1, Add/1
  knee pos & vel/1 -> Demux1/1, Demux3/1
  Subsystem/1(T_spring) -> To Workspace3/1, Add/2

== system Leg_Sim_VariableDamping/system/permutations ==
  q : Inport
  qd : Inport  Port=2
  qdd : Inport  Port=3
  "tau " : Inport  Port=4
  Integrator : Integrator
  Mux : Mux  Inputs=2
  Product1 : Product
  To Workspace1 : ToWorkspace  VariableName=qd  SampleTime=-1
      settings: Save2DSignal=2-D array (concatenate along first dimension)
  To Workspace13 : ToWorkspace  VariableName=tau  SampleTime=-1
      settings: Save2DSignal=2-D array (concatenate along first dimension)
  To Workspace14 : ToWorkspace  VariableName=qdd  SampleTime=-1
      settings: Save2DSignal=2-D array (concatenate along first dimension)
  To Workspace15 : ToWorkspace  VariableName=E_joint  SampleTime=-1
      settings: Save2DSignal=2-D array (concatenate along first dimension)
  To Workspace4 : ToWorkspace  VariableName=q  SampleTime=-1
      settings: Save2DSignal=2-D array (concatenate along first dimension)
  tau : Outport
  pos & vel : Outport  Port=2
  wires:
  qd/1 -> Mux/2, Product1/1, To Workspace1/1
  Integrator/1 -> To Workspace15/1
  "tau "/1 -> tau/1, To Workspace13/1, Product1/2
  q/1 -> Mux/1, To Workspace4/1
  Product1/1 -> Integrator/1
  qdd/1 -> To Workspace14/1
  Mux/1 -> pos & vel/1

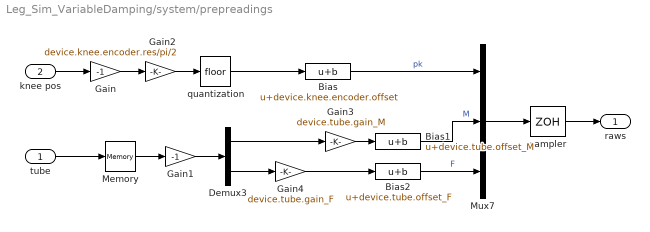
== system Leg_Sim_VariableDamping/system/prepreadings ==
  tube : Inport
  knee pos : Inport  Port=2
  Bias : Bias  Bias=device.knee.encoder.offset
  Bias1 : Bias  Bias=device.tube.offset_M
  Bias2 : Bias  Bias=device.tube.offset_F
  Demux3 : Demux  Outputs=2
  Gain : Gain  Gain=-1
  Gain1 : Gain  Gain=-1
  Gain2 : Gain  Gain=device.knee.encoder.res/pi/2
  Gain3 : Gain  Gain=device.tube.gain_M
  Gain4 : Gain  Gain=device.tube.gain_F
  Memory : Memory
  Mux7 : Mux  Inputs=3
  quantization : Rounding
  sampler : ZeroOrderHold  SampleTime=ctrl.t_step
  raws : Outport
  wires:
  Gain2/1 -> quantization/1
  Bias1/1 -> Mux7/2  "M"
  Gain1/1 -> Demux3/1
  Gain3/1 -> Bias1/1
  Demux3/1 -> Gain3/1
  Bias2/1 -> Mux7/3  "F"
  Gain4/1 -> Bias2/1
  Memory/1 -> Gain1/1
  Mux7/1 -> sampler/1
  sampler/1 -> raws/1
  Gain/1 -> Gain2/1
  tube/1 -> Memory/1
  knee pos/1 -> Gain/1
  Demux3/2 -> Gain4/1
  quantization/1 -> Bias/1
  Bias/1 -> Mux7/1  "pk"

== system Leg_Sim_VariableDamping/ctrl/Signal processing/low-pass ==
  x : Inport
  C : Constant  Value=tan(pi*Wn/2)
  Dot Product : DotProduct  InputSameDT=on  OutDataTypeStr=Inherit: Inherit via internal rule
  Fcn : Fcn  Expr=u/(u+1)
  Fcn1 : Fcn  Expr=(1-u)/(u+1)
  Mux : Mux  Inputs=3
  Mux1 : Mux  Inputs=3
  x-1 : UnitDelay  Description=Store in Global RAM  DisableCoverage=on  SampleTime=-1  HasFrameUpgradeWarning=on
  y-1 : UnitDelay  Description=Store in Global RAM  DisableCoverage=on  SampleTime=-1  HasFrameUpgradeWarning=on
  y : Outport
  wires:
  x/1 -> Mux1/1, x-1/1
  y-1/1 -> Mux1/3
  C/1 -> Fcn1/1, Fcn/1
  Fcn/1 -> Mux/2, Mux/1
  Fcn1/1 -> Mux/3
  Mux1/1 -> Dot Product/2
  Mux/1 -> Dot Product/1
  Dot Product/1 -> y-1/1, y/1
  x-1/1 -> Mux1/2

== system Leg_Sim_VariableDamping/system/HDgc/merge fd&id q ==
  in1 : Inport
  in2 : Inport  Port=2
  Assignment3 : Assignment  DiagnosticForDimensions=Warning  IndexOptions=Index vector (dialog)  Indices=i_id  OutputSizes=1
  Assignment4 : Assignment  DiagnosticForDimensions=Warning  IndexOptions=Index vector (dialog)  Indices=i_fd  OutputSizes=1
  zeros : Constant  Value=zeros(model.NB,1)
  out : Outport
  wires:
  in2/1 -> Assignment3/2
  in1/1 -> Assignment4/2
  Assignment3/1 -> out/1
  Assignment4/1 -> Assignment3/1
  zeros/1 -> Assignment4/1

== system Leg_Sim_VariableDamping/system/HDgc/merge fd&id qd ==
  in1 : Inport
  in2 : Inport  Port=2
  Assignment3 : Assignment  DiagnosticForDimensions=Warning  IndexOptions=Index vector (dialog)  Indices=i_id  OutputSizes=1
  Assignment4 : Assignment  DiagnosticForDimensions=Warning  IndexOptions=Index vector (dialog)  Indices=i_fd  OutputSizes=1
  zeros : Constant  Value=zeros(model.NB,1)
  out : Outport
  wires:
  zeros/1 -> Assignment4/1
  Assignment4/1 -> Assignment3/1
  Assignment3/1 -> out/1
  in1/1 -> Assignment4/2
  in2/1 -> Assignment3/2

== system Leg_Sim_VariableDamping/system/HDgc/merge fd&id qdd ==
  in1 : Inport
  in2 : Inport  Port=2
  Assignment3 : Assignment  DiagnosticForDimensions=Warning  IndexOptions=Index vector (dialog)  Indices=i_id  OutputSizes=1
  Assignment4 : Assignment  DiagnosticForDimensions=Warning  IndexOptions=Index vector (dialog)  Indices=i_fd  OutputSizes=1
  zeros : Constant  Value=zeros(model.NB,1)
  out : Outport
  wires:
  zeros/1 -> Assignment4/1
  Assignment4/1 -> Assignment3/1
  Assignment3/1 -> out/1
  in1/1 -> Assignment4/2
  in2/1 -> Assignment3/2

== system Leg_Sim_VariableDamping/system/HDgc/merge fd&id tau ==
  in1 : Inport
  in2 : Inport  Port=2
  Assignment3 : Assignment  DiagnosticForDimensions=Warning  IndexOptions=Index vector (dialog)  Indices=i_id  OutputSizes=1
  Assignment4 : Assignment  DiagnosticForDimensions=Warning  IndexOptions=Index vector (dialog)  Indices=i_fd  OutputSizes=1
  zeros : Constant  Value=zeros(model.NB,1)
  out : Outport
  wires:
  in2/1 -> Assignment3/2
  in1/1 -> Assignment4/2
  Assignment3/1 -> out/1
  Assignment4/1 -> Assignment3/1
  zeros/1 -> Assignment4/1

== system Leg_Sim_VariableDamping/system/ankle prosthesis model/spring damper ==
  x : Inport
  xd : Inport  Port=2
  Gain4 : Gain  Gain=ank.k
  Gain8 : Gain  Gain=ank.c
  Gain9 : Gain  Gain=1/2
  Integrator : Integrator
  Mux1 : Mux  Inputs=2
  Product1 : Product
  Product2 : Product
  Sum2 : Sum  Inputs=|--
  F : Outport
  E : Outport  Port=2
  wires:
  Product2/1 -> Integrator/1
  Gain4/1 -> Sum2/1, Product1/2
  Gain8/1 -> Sum2/2, Product2/1
  xd/1 -> Product2/2, Gain8/1
  x/1 -> Product1/1, Gain4/1
  Product1/1 -> Gain9/1
  Sum2/1 -> F/1
  Integrator/1 -> Mux1/2
  Gain9/1 -> Mux1/1
  Mux1/1 -> E/1

== system Leg_Sim_VariableDamping/system/human model/Subsystem4 ==
  qcmd : Inport
  delay : Inport  Port=2
  Demux : Demux
  Mux : Mux
  Mux1 : Mux
  Mux2 : Mux
  Subsystem1 : Subsystem  mask{Z_DR=ref.Z_DR, y0=q0(2), yd0=qd0(2)}
      mask prompts: Z_DR "controller damping ratio"; y0 "initial condition position"; yd0 "initial condition velocity"
  Subsystem2 : Subsystem  mask{Z_DR=ref.Z_DR, y0=q0(1), yd0=qd0(1)}
      mask prompts: Z_DR "controller damping ratio"; y0 "initial condition position"; yd0 "initial condition velocity"
  Subsystem3 : Subsystem  mask{Z_DR=ref.Z_DR, y0=q0(3), yd0=qd0(3)}
      mask prompts: Z_DR "controller damping ratio"; y0 "initial condition position"; yd0 "initial condition velocity"
  Subsystem4 : Subsystem  mask{Z_DR=ref.Z_DR, y0=q0(4), yd0=qd0(4)}
      mask prompts: Z_DR "controller damping ratio"; y0 "initial condition position"; yd0 "initial condition velocity"
  Sum : Sum  Inputs=-+|
  qref : Outport  OutDataTypeStr=double  PortDimensions=4
  qdref : Outport  Port=2  OutDataTypeStr=double  PortDimensions=4
  qddref : Outport  Port=3  OutDataTypeStr=double  PortDimensions=4
  wires:
  delay/1 -> Subsystem4/2(t_delay), Subsystem3/2(t_delay), Subsystem1/2(t_delay), Subsystem2/2(t_delay)
  Sum/1 -> Subsystem4/1(ycmd)
  Demux/4 -> Sum/2
  Demux/2 -> Subsystem1/1(ycmd)
  Demux/1 -> Subsystem2/1(ycmd)
  qcmd/1 -> Demux/1
  Demux/3 -> Sum/1, Subsystem3/1(ycmd)
  Subsystem1/2(ydref) -> Mux1/2
  Subsystem2/1(yref) -> Mux/1
  Subsystem1/1(yref) -> Mux/2
  Subsystem3/1(yref) -> Mux/3
  Subsystem4/1(yref) -> Mux/4
  Subsystem2/2(ydref) -> Mux1/1
  Subsystem3/2(ydref) -> Mux1/3
  Subsystem4/2(ydref) -> Mux1/4
  Mux1/1 -> qdref/1
  Mux/1 -> qref/1
  Subsystem2/3(yddref) -> Mux2/1
  Subsystem1/3(yddref) -> Mux2/2
  Subsystem3/3(yddref) -> Mux2/3
  Subsystem4/3(yddref) -> Mux2/4
  Mux2/1 -> qddref/1

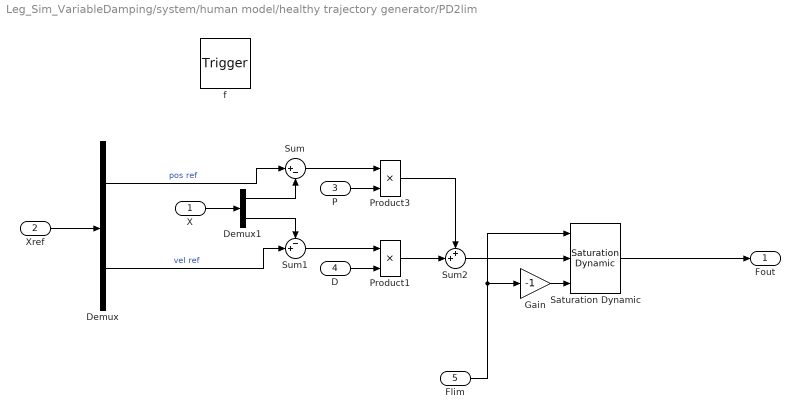
== system Leg_Sim_VariableDamping/system/human model/healthy trajectory generator/PD2lim ==
  X : Inport  OutDataTypeStr=double  PortDimensions=[1 2]
  Xref : Inport  Port=2  OutDataTypeStr=double  PortDimensions="[1  2]"
  P : Inport  Port=3  OutDataTypeStr=double  PortDimensions=1
  D : Inport  Port=4  OutDataTypeStr=double  PortDimensions=1
  Flim : Inport  Port=5  OutDataTypeStr=double  PortDimensions=1
  f : TriggerPort  TriggerType=function-call  VariantControl=(inherit)
      settings: CopyFcn=Stateflow.SLINSF.SimulinkMan.removeBlockPreDeleteFcn  PreDeleteFcn=Stateflow.SLINSF.SimulinkMan.unsafePredeleteFcn
  Demux : Demux  Outputs=2
  Demux1 : Demux  Outputs=2
  Gain : Gain  Gain=-1
  Product1 : Product
  Product3 : Product
  Saturation Dynamic : simulink/Discontinuities/Saturation Dynamic  OutMin=[]  OutMax=[]  OutDataTypeStr=Inherit: Same as second input  OutDataType=fixdt(1, 16)  OutScaling=2^-10  DoSatur=off
  Sum : Sum  Inputs=|+-
  Sum1 : Sum  Inputs=-+|
  Sum2 : Sum  Inputs=++|
  Fout : Outport  PortDimensions=1
  wires:
  Product1/1 -> Sum2/2
  Product3/1 -> Sum2/1
  Demux1/2 -> Sum1/1
  Sum/1 -> Product3/1
  Demux/2 -> Sum1/2  "vel ref"
  Sum1/1 -> Product1/1
  Demux/1 -> Sum/1  "pos ref"
  Xref/1 -> Demux/1
  P/1 -> Product3/2
  D/1 -> Product1/2
  Demux1/1 -> Sum/2
  X/1 -> Demux1/1
  Sum2/1 -> Saturation Dynamic/2
  Saturation Dynamic/1 -> Fout/1
  Gain/1 -> Saturation Dynamic/3
  Flim/1 -> Gain/1, Saturation Dynamic/1

== system Leg_Sim_VariableDamping/system/knee prosthesis model/Subsystem ==
  pos : Inport
  Divide2 : Product
  Gain7 : Gain  Gain=-dmp.k
  Gain8 : Gain  Gain=-1/2
  To Workspace9 : ToWorkspace  VariableName=E_ps  SampleTime=-1
      settings: Save2DSignal=2-D array (concatenate along first dimension)
  T_spring : Outport
  wires:
  pos/1 -> Gain7/1, Gain8/1
  Divide2/1 -> To Workspace9/1
  Gain7/1 -> T_spring/1, Divide2/2
  Gain8/1 -> Divide2/1

== system Leg_Sim_VariableDamping/system/knee prosthesis model/Subsystem1 ==
  note: All direction gains are +1 for a lower limit
      | and -1 for an upper limit.  In effect, upper
      | limits are mapped onto lower limits.
  x : Inport
  xd : Inport  Port=2
  Bias : Bias  Bias=-pos
  Energy Audit : Subsystem
  If : If  IfExpression=u1<0  ShowElse=off
  If Action Subsystem : Subsystem  TreatAsAtomicUnit=on
  dir x : Gain  Gain=3-2*dir
  F : Outport
  E : Outport  Port=2  VectorParamsAs1DForOutWhenUnconnected=off
  wires:
  dir x/1 -> If Action Subsystem/1(xrel), If/1
  x/1 -> Bias/1
  If/1 -> If Action Subsystem/Action
  xd/1 -> Energy Audit/4(dx), If Action Subsystem/2(xd)
  If Action Subsystem/1(F) -> Energy Audit/1(F), F/1
  Bias/1 -> dir x/1
  If Action Subsystem/2(Ps) -> Energy Audit/2(P_spring)  "P_spring"
  If Action Subsystem/3(Es) -> Energy Audit/3(E_spring)  "E_spring"
  Energy Audit/1(E) -> E/1

== system Leg_Sim_VariableDamping/system/knee prosthesis model/Subsystem2 ==
  note: All direction gains are +1 for a lower limit
      | and -1 for an upper limit.  In effect, upper
      | limits are mapped onto lower limits.
  x : Inport
  xd : Inport  Port=2
  Bias : Bias  Bias=-pos
  Energy Audit : Subsystem
  If : If  IfExpression=u1<0  ShowElse=off
  If Action Subsystem : Subsystem  TreatAsAtomicUnit=on
  dir x : Gain  Gain=3-2*dir
  F : Outport
  E : Outport  Port=2  VectorParamsAs1DForOutWhenUnconnected=off
  wires:
  Energy Audit/1(E) -> E/1
  If Action Subsystem/3(Es) -> Energy Audit/3(E_spring)  "E_spring"
  If Action Subsystem/2(Ps) -> Energy Audit/2(P_spring)  "P_spring"
  Bias/1 -> dir x/1
  If Action Subsystem/1(F) -> F/1, Energy Audit/1(F)
  xd/1 -> If Action Subsystem/2(xd), Energy Audit/4(dx)
  If/1 -> If Action Subsystem/Action
  x/1 -> Bias/1
  dir x/1 -> If/1, If Action Subsystem/1(xrel)

== system Leg_Sim_VariableDamping/system/knee prosthesis model/minimum damping//friction ==
  speed : Inport
  Add1 : Sum
  Atan : Trigonometry  Operator=tanh
  Gain1 : Gain  Gain=-dmp.c
  Gain4 : Gain  Gain=100
  Gain5 : Gain  Gain=-dmp.T_stic
  Integrator1 : Integrator
  Integrator2 : Integrator
  Product4 : Product
  Product5 : Product
  Sum : Sum  Inputs=|++
  To Workspace2 : ToWorkspace  VariableName=E_fric  SampleTime=-1
      settings: Save2DSignal=2-D array (concatenate along first dimension)
  T_fric : Outport
  wires:
  Product5/1 -> Integrator2/1
  Product4/1 -> Integrator1/1
  speed/1 -> Gain1/1, Product5/2, Product4/2, Gain4/1
  Gain1/1 -> Product4/1, Sum/1
  Integrator2/1 -> Add1/2
  Integrator1/1 -> Add1/1
  Gain5/1 -> Product5/1, Sum/2
  Atan/1 -> Gain5/1
  Gain4/1 -> Atan/1
  Add1/1 -> To Workspace2/1
  Sum/1 -> T_fric/1

== system Leg_Sim_VariableDamping/system/knee prosthesis model/regulated quadratic damping ==
  c : Inport
  speed : Inport  Port=2
  Abs : Abs  ZeroCross=off
  Gain3 : Gain  Gain=-1
  Product2 : Product
  Product3 : Product
  T_act : Outport
  wires:
  Product2/1 -> T_act/1
  speed/1 -> Abs/1, Product3/2
  Product3/1 -> Product2/1
  Gain3/1 -> Product3/1
  c/1 -> Gain3/1
  Abs/1 -> Product2/2

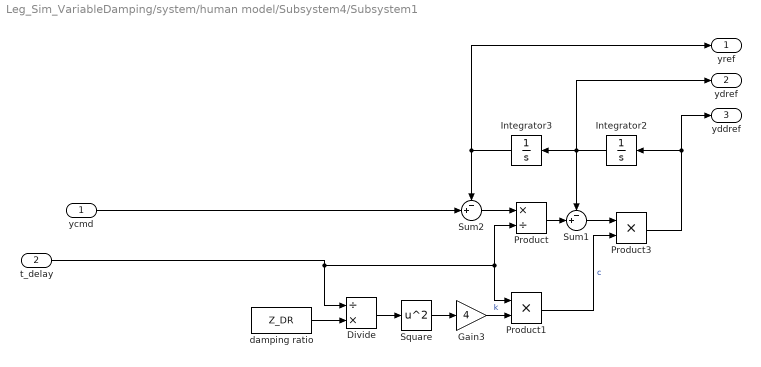
== system Leg_Sim_VariableDamping/system/human model/Subsystem4/Subsystem1 ==
  ycmd : Inport
  t_delay : Inport  Port=2
  Divide : Product  Inputs=/*
  Gain3 : Gain  Gain=4
  Integrator2 : Integrator  InitialCondition=yd0
  Integrator3 : Integrator  InitialCondition=y0
  Product : Product  Inputs=*/
  Product1 : Product
  Product3 : Product
  Square : Math  Operator=square  SaturateOnIntegerOverflow=on
  Sum1 : Sum  Inputs=-+|
  Sum2 : Sum  Inputs=-+|
  damping ratio : Constant  Value=Z_DR
  yref : Outport  PortDimensions=1
  ydref : Outport  Port=2  PortDimensions=1
  yddref : Outport  Port=3  PortDimensions=1
  wires:
  Integrator3/1 -> Sum2/1, yref/1
  Integrator2/1 -> Integrator3/1, Sum1/1, ydref/1
  t_delay/1 -> Divide/1, Product1/1, Product/2
  Product3/1 -> Integrator2/1, yddref/1
  Product/1 -> Sum1/2
  Square/1 -> Gain3/1
  ycmd/1 -> Sum2/2
  Product1/1 -> Product3/2  "c"
  Gain3/1 -> Product1/2  "k"
  Sum1/1 -> Product3/1
  Sum2/1 -> Product/1
  Divide/1 -> Square/1
  damping ratio/1 -> Divide/2

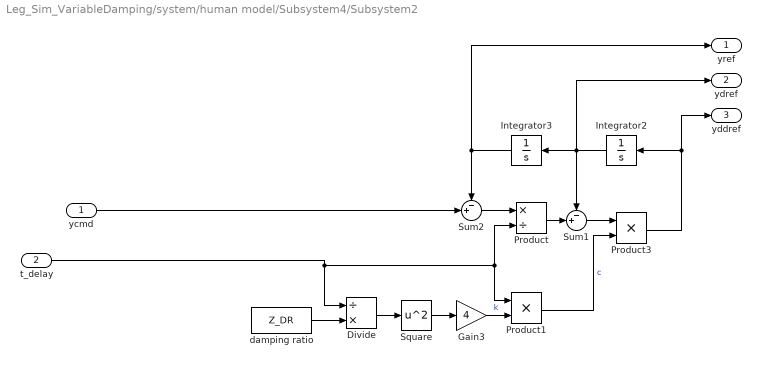
== system Leg_Sim_VariableDamping/system/human model/Subsystem4/Subsystem2 ==
  ycmd : Inport
  t_delay : Inport  Port=2
  Divide : Product  Inputs=/*
  Gain3 : Gain  Gain=4
  Integrator2 : Integrator  InitialCondition=yd0
  Integrator3 : Integrator  InitialCondition=y0
  Product : Product  Inputs=*/
  Product1 : Product
  Product3 : Product
  Square : Math  Operator=square  SaturateOnIntegerOverflow=on
  Sum1 : Sum  Inputs=-+|
  Sum2 : Sum  Inputs=-+|
  damping ratio : Constant  Value=Z_DR
  yref : Outport  PortDimensions=1
  ydref : Outport  Port=2  PortDimensions=1
  yddref : Outport  Port=3  PortDimensions=1
  wires:
  damping ratio/1 -> Divide/2
  Divide/1 -> Square/1
  Sum2/1 -> Product/1
  Sum1/1 -> Product3/1
  Gain3/1 -> Product1/2  "k"
  Product1/1 -> Product3/2  "c"
  ycmd/1 -> Sum2/2
  Square/1 -> Gain3/1
  Product/1 -> Sum1/2
  Product3/1 -> yddref/1, Integrator2/1
  t_delay/1 -> Product/2, Product1/1, Divide/1
  Integrator2/1 -> ydref/1, Sum1/1, Integrator3/1
  Integrator3/1 -> yref/1, Sum2/1

== system Leg_Sim_VariableDamping/system/human model/Subsystem4/Subsystem3 ==
  ycmd : Inport
  t_delay : Inport  Port=2
  Divide : Product  Inputs=/*
  Gain3 : Gain  Gain=4
  Integrator2 : Integrator  InitialCondition=yd0
  Integrator3 : Integrator  InitialCondition=y0
  Product : Product  Inputs=*/
  Product1 : Product
  Product3 : Product
  Square : Math  Operator=square  SaturateOnIntegerOverflow=on
  Sum1 : Sum  Inputs=-+|
  Sum2 : Sum  Inputs=-+|
  damping ratio : Constant  Value=Z_DR
  yref : Outport  PortDimensions=1
  ydref : Outport  Port=2  PortDimensions=1
  yddref : Outport  Port=3  PortDimensions=1
  wires:
  damping ratio/1 -> Divide/2
  Divide/1 -> Square/1
  Sum2/1 -> Product/1
  Sum1/1 -> Product3/1
  Gain3/1 -> Product1/2  "k"
  Product1/1 -> Product3/2  "c"
  ycmd/1 -> Sum2/2
  Square/1 -> Gain3/1
  Product/1 -> Sum1/2
  Product3/1 -> yddref/1, Integrator2/1
  t_delay/1 -> Product/2, Product1/1, Divide/1
  Integrator2/1 -> ydref/1, Sum1/1, Integrator3/1
  Integrator3/1 -> yref/1, Sum2/1

== system Leg_Sim_VariableDamping/system/human model/Subsystem4/Subsystem4 ==
  ycmd : Inport
  t_delay : Inport  Port=2
  Divide : Product  Inputs=/*
  Gain3 : Gain  Gain=4
  Integrator2 : Integrator  InitialCondition=yd0
  Integrator3 : Integrator  InitialCondition=y0
  Product : Product  Inputs=*/
  Product1 : Product
  Product3 : Product
  Square : Math  Operator=square  SaturateOnIntegerOverflow=on
  Sum1 : Sum  Inputs=-+|
  Sum2 : Sum  Inputs=-+|
  damping ratio : Constant  Value=Z_DR
  yref : Outport  PortDimensions=1
  ydref : Outport  Port=2  PortDimensions=1
  yddref : Outport  Port=3  PortDimensions=1
  wires:
  Integrator3/1 -> Sum2/1, yref/1
  Integrator2/1 -> Integrator3/1, Sum1/1, ydref/1
  t_delay/1 -> Divide/1, Product1/1, Product/2
  Product3/1 -> Integrator2/1, yddref/1
  Product/1 -> Sum1/2
  Square/1 -> Gain3/1
  ycmd/1 -> Sum2/2
  Product1/1 -> Product3/2  "c"
  Gain3/1 -> Product1/2  "k"
  Sum1/1 -> Product3/1
  Sum2/1 -> Product/1
  Divide/1 -> Square/1
  damping ratio/1 -> Divide/2

== system Leg_Sim_VariableDamping/system/knee prosthesis model/Subsystem1/Energy Audit ==
  F : Inport
  P_spring : Inport  Port=2
  E_spring : Inport  Port=3
  dx : Inport  Port=4
  Bus Creator : BusCreator  Inputs=4
  Integrator : Integrator
  Product : Product
  Sum : Sum  Inputs=--|
  E : Outport
  wires:
  Bus Creator/1 -> E/1
  E_spring/1 -> Bus Creator/2
  P_spring/1 -> Sum/1, Bus Creator/1
  dx/1 -> Product/2
  F/1 -> Product/1
  Product/1 -> Sum/2
  Sum/1 -> Integrator/1, Bus Creator/3
  Integrator/1 -> Bus Creator/4

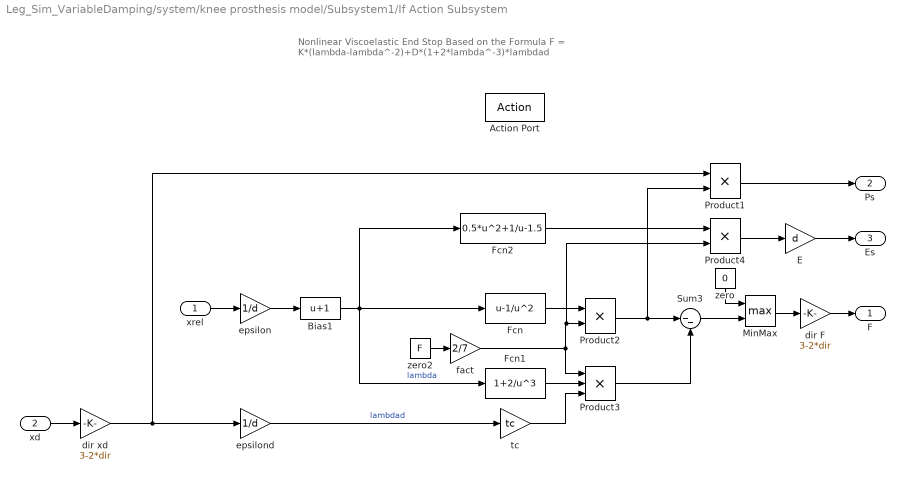
== system Leg_Sim_VariableDamping/system/knee prosthesis model/Subsystem1/If Action Subsystem ==
  note: Nonlinear Viscoelastic End Stop Based on the Formula F = K*(lambda-lambda^-2)+D*(1+2*lambda^-3)*lambdad
  xrel : Inport
  xd : Inport  Port=2
  Action Port : ActionPort  ActionPortLabel=if(u1<0)
  Bias1 : Bias  Bias=1
  E : Gain  Gain=d
  Fcn : Fcn  Expr=u-1/u^2
  Fcn1 : Fcn  Expr=1+2/u^3
  Fcn2 : Fcn  Expr=0.5*u^2+1/u-1.5
  MinMax : MinMax  Function=max  Inputs=2
  Product1 : Product
  Product2 : Product
  Product3 : Product  Inputs=3
  Product4 : Product
  Sum3 : Sum  Inputs=|--
  dir F : Gain  Gain=3-2*dir
  dir xd : Gain  Gain=3-2*dir
  epsilon : Gain  Gain=1/d
  epsilond : Gain  Gain=1/d
  fact : Gain  Gain=2/7
  tc : Gain  Gain=tc
  zero : Constant  Value=0
  zero2 : Constant  Value=F
  F : Outport
  Ps : Outport  Port=2
  Es : Outport  Port=3
  wires:
  dir F/1 -> F/1
  tc/1 -> Product3/3
  Product3/1 -> Sum3/2
  Bias1/1 -> Fcn1/1, Fcn2/1, Fcn/1  "lambda"
  fact/1 -> Product4/2, Product2/2, Product3/1
  Fcn1/1 -> Product3/2
  Product2/1 -> Product1/2, Sum3/1
  Fcn/1 -> Product2/1
  zero/1 -> MinMax/1
  MinMax/1 -> dir F/1
  zero2/1 -> fact/1
  Sum3/1 -> MinMax/2
  xd/1 -> dir xd/1
  epsilond/1 -> tc/1  "lambdad"
  epsilon/1 -> Bias1/1
  xrel/1 -> epsilon/1
  Product1/1 -> Ps/1
  dir xd/1 -> Product1/1, epsilond/1
  Product4/1 -> E/1
  E/1 -> Es/1
  Fcn2/1 -> Product4/1

== system Leg_Sim_VariableDamping/system/knee prosthesis model/Subsystem2/Energy Audit ==
  F : Inport
  P_spring : Inport  Port=2
  E_spring : Inport  Port=3
  dx : Inport  Port=4
  Bus Creator : BusCreator  Inputs=4
  Integrator : Integrator
  Product : Product
  Sum : Sum  Inputs=--|
  E : Outport
  wires:
  Integrator/1 -> Bus Creator/4
  Sum/1 -> Bus Creator/3, Integrator/1
  Product/1 -> Sum/2
  F/1 -> Product/1
  dx/1 -> Product/2
  P_spring/1 -> Bus Creator/1, Sum/1
  E_spring/1 -> Bus Creator/2
  Bus Creator/1 -> E/1

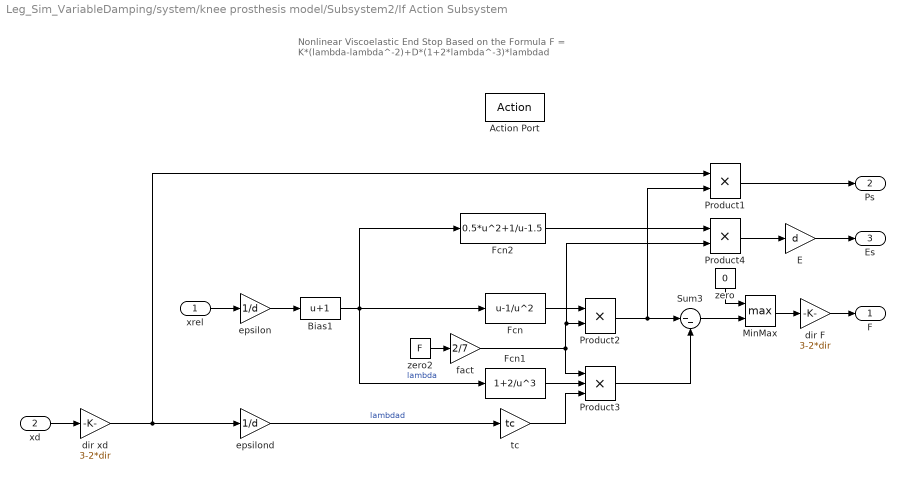
== system Leg_Sim_VariableDamping/system/knee prosthesis model/Subsystem2/If Action Subsystem ==
  note: Nonlinear Viscoelastic End Stop Based on the Formula F = K*(lambda-lambda^-2)+D*(1+2*lambda^-3)*lambdad
  xrel : Inport
  xd : Inport  Port=2
  Action Port : ActionPort  ActionPortLabel=if(u1<0)
  Bias1 : Bias  Bias=1
  E : Gain  Gain=d
  Fcn : Fcn  Expr=u-1/u^2
  Fcn1 : Fcn  Expr=1+2/u^3
  Fcn2 : Fcn  Expr=0.5*u^2+1/u-1.5
  MinMax : MinMax  Function=max  Inputs=2
  Product1 : Product
  Product2 : Product
  Product3 : Product  Inputs=3
  Product4 : Product
  Sum3 : Sum  Inputs=|--
  dir F : Gain  Gain=3-2*dir
  dir xd : Gain  Gain=3-2*dir
  epsilon : Gain  Gain=1/d
  epsilond : Gain  Gain=1/d
  fact : Gain  Gain=2/7
  tc : Gain  Gain=tc
  zero : Constant  Value=0
  zero2 : Constant  Value=F
  F : Outport
  Ps : Outport  Port=2
  Es : Outport  Port=3
  wires:
  Fcn2/1 -> Product4/1
  E/1 -> Es/1
  Product4/1 -> E/1
  dir xd/1 -> epsilond/1, Product1/1
  Product1/1 -> Ps/1
  xrel/1 -> epsilon/1
  epsilon/1 -> Bias1/1
  epsilond/1 -> tc/1  "lambdad"
  xd/1 -> dir xd/1
  Sum3/1 -> MinMax/2
  zero2/1 -> fact/1
  MinMax/1 -> dir F/1
  zero/1 -> MinMax/1
  Fcn/1 -> Product2/1
  Product2/1 -> Sum3/1, Product1/2
  Fcn1/1 -> Product3/2
  fact/1 -> Product3/1, Product2/2, Product4/2
  Bias1/1 -> Fcn/1, Fcn2/1, Fcn1/1  "lambda"
  Product3/1 -> Sum3/2
  tc/1 -> Product3/3
  dir F/1 -> F/1
